simulink model "problema2"  (R2021b)
settings: Solver=VariableStepAuto  StartTime=0.0  StopTime=10.0  RelTol=1e-3
undefined symbols (not defined in the file or in its folder): A, B, C, D
libraries: simulink x2
settings Model: Creator=laurentiu  LastModifiedBy=laurentiu

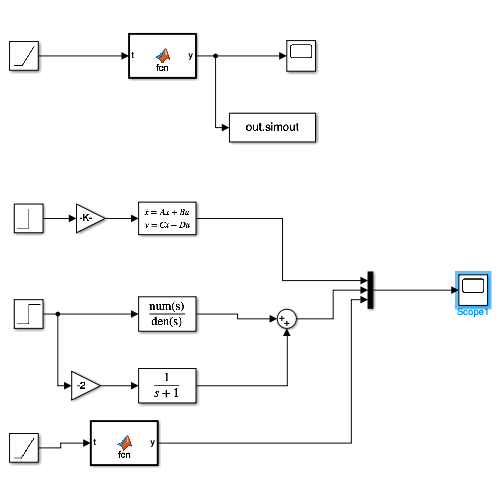
[thumbnail: Simulink's stored preview of the top-level diagram]
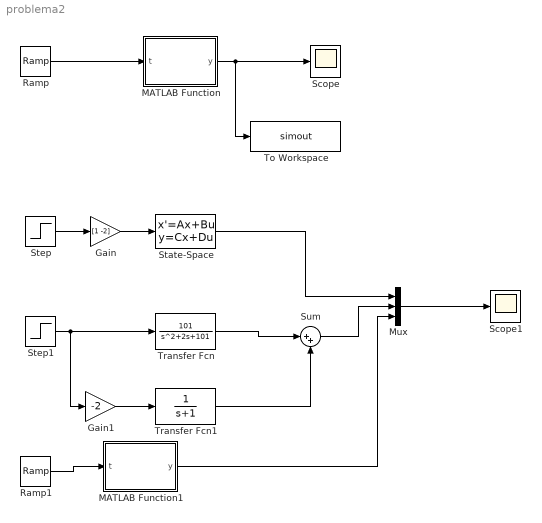
== system problema2 ==
  Gain : Gain  Gain=[1 -2]
  Gain1 : Gain  Gain=-2
  MATLAB Function : MATLAB Function  TreatAsAtomicUnit=on
  MATLAB Function1 : MATLAB Function  TreatAsAtomicUnit=on
  Mux : Mux  Inputs=3
  Ramp : simulink/Sources/Ramp  slope=1  start=0  InitialOutput=0
  Ramp1 : simulink/Sources/Ramp  slope=1  start=0  InitialOutput=0
  Scope : Scope
  Scope1 : Scope
  State-Space : StateSpace  A=A  B=B  C=C  D=D  InitialCondition=0
  Step : Step  Time=0  SampleTime=0
  Step1 : Step  Time=0  SampleTime=0
  Sum : Sum  Inputs=|++
  To Workspace : ToWorkspace  VariableName=simout  SaveFormat=Timeseries  SampleTime=-1
  Transfer Fcn : TransferFcn  Numerator=[0 0 101]  Denominator=[1, 2, 101]
  Transfer Fcn1 : TransferFcn  Denominator=[1 1]
  wires:
  Ramp/1 -> MATLAB Function/1(t)
  MATLAB Function/1(y) -> To Workspace/1, Scope/1
  Step/1 -> Gain/1
  Gain/1 -> State-Space/1
  Step1/1 -> Gain1/1, Transfer Fcn/1
  State-Space/1 -> Mux/1
  Transfer Fcn/1 -> Sum/1
  Transfer Fcn1/1 -> Sum/2
  Sum/1 -> Mux/2
  Ramp1/1 -> MATLAB Function1/1(t)
  MATLAB Function1/1(y) -> Mux/3
  Mux/1 -> Scope1/1
  Gain1/1 -> Transfer Fcn1/1

== matlab function problema2/MATLAB Function ==
  data: t input; y output
function y = fcn(t)

y = exp(-t) - 101*exp(-t)*(cos(10*t) + sin(10*t)/10) + (101*sin(10*t)*exp(-t))/10;

== matlab function problema2/MATLAB Function1 ==
  data: t input; y output
function y = fcn(t)

y = 2*exp(-t) - exp(-t)*(cos(10*t) + sin(10*t)/10) - 1;
